simulink model "ekf_trial"  (Simulink 8.1)
settings: Solver=ode45  StartTime=0.0  StopTime=500  FixedStep=0.5  MaxStep=0.01  RelTol=1e-3
values from neighbouring files (symbols this model uses):
  A = [SUN_COPY_X,SUN_COPY_Y,SUN_COPY_Z]    [returnNormalsAndFluxes.m]
  B = [0,1,0]    [returnNormalsAndFluxes.m]
  R = [new_x;new_y;new_z]    [FINAL_PROGRAM.m]    (also in Graphical_Calculation.m; optimizedCalculation.m; optimizedCalculation_FINAL.m; returnNormalsAndFluxes.m)
undefined symbols (not defined in the file or in its folder): Ad, Bd, C, dt, L, P0_guess, Q, x0, x0_guess
settings Model: Creator=Sumeet Singh  LastModifiedBy=DJackson
settings SolverCC: ZcThreshold=1e-8  ZeroCrossControl=EnableAll  ZeroCrossAlgorithm=Adaptive
settings DataIOCC: ExternalInput=tu  LimitDataPoints=off
settings DebuggingCC: SolverPrmCheckMsg=none
settings SFSimCC: SimParseCustomCode=off

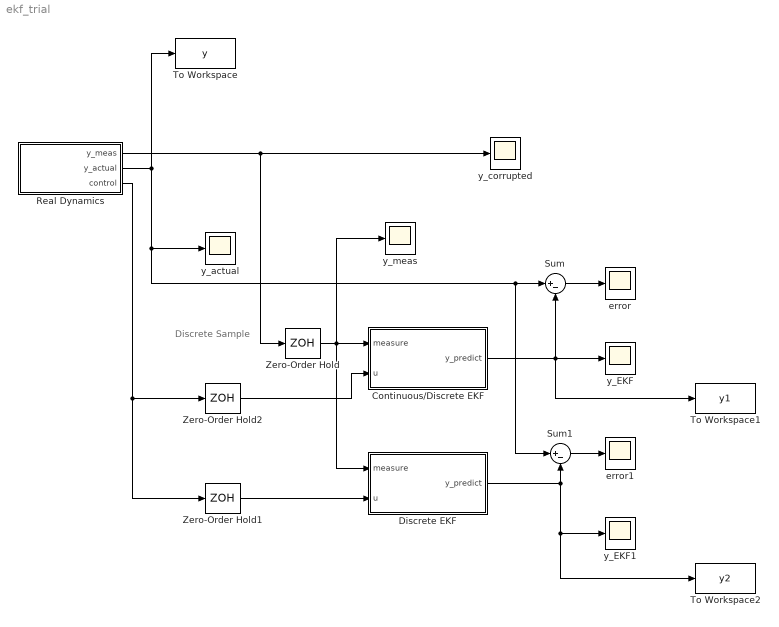
== system ekf_trial ==
  note: Discrete Sample
  Continuous/Discrete EKF : Subsystem
  Discrete EKF : Subsystem
  "Real Dynamics " : Subsystem
  Sum : Sum  Inputs=|+-
  Sum1 : Sum  Inputs=|+-
  To Workspace : ToWorkspace  VariableName=y  SampleTime=dt
  To Workspace1 : ToWorkspace  VariableName=y1  SampleTime=dt
  To Workspace2 : ToWorkspace  VariableName=y2  SampleTime=dt
  Zero-Order Hold : ZeroOrderHold  SampleTime=dt
  Zero-Order Hold1 : ZeroOrderHold  SampleTime=dt
  Zero-Order Hold2 : ZeroOrderHold  SampleTime=dt
  error : Scope
      settings: SaveName=ScopeData5
  error1 : Scope
      settings: SaveName=ScopeData6
  y_EKF : Scope
      settings: SaveName=ScopeData2
  y_EKF1 : Scope
      settings: SaveName=ScopeData8
  y_actual : Scope
  y_corrupted : Scope
  y_meas : Scope
      settings: SaveName=ScopeData4
  wires:
  Continuous/Discrete EKF/1(y_predict) -> To Workspace1/1, Sum/2, y_EKF/1
  "Real Dynamics "/3(control) -> Zero-Order Hold2/1, Zero-Order Hold1/1
  "Real Dynamics "/1(y_meas) -> y_corrupted/1, Zero-Order Hold/1
  "Real Dynamics "/2(y_actual) -> Sum1/1, Sum/1, y_actual/1, To Workspace/1
  Sum/1 -> error/1
  Zero-Order Hold1/1 -> Discrete EKF/2(u)
  Zero-Order Hold/1 -> Continuous/Discrete EKF/1(measure), y_meas/1, Discrete EKF/1(measure)
  Discrete EKF/1(y_predict) -> To Workspace2/1, y_EKF1/1, Sum1/2
  Sum1/1 -> error1/1
  Zero-Order Hold2/1 -> Continuous/Discrete EKF/2(u)

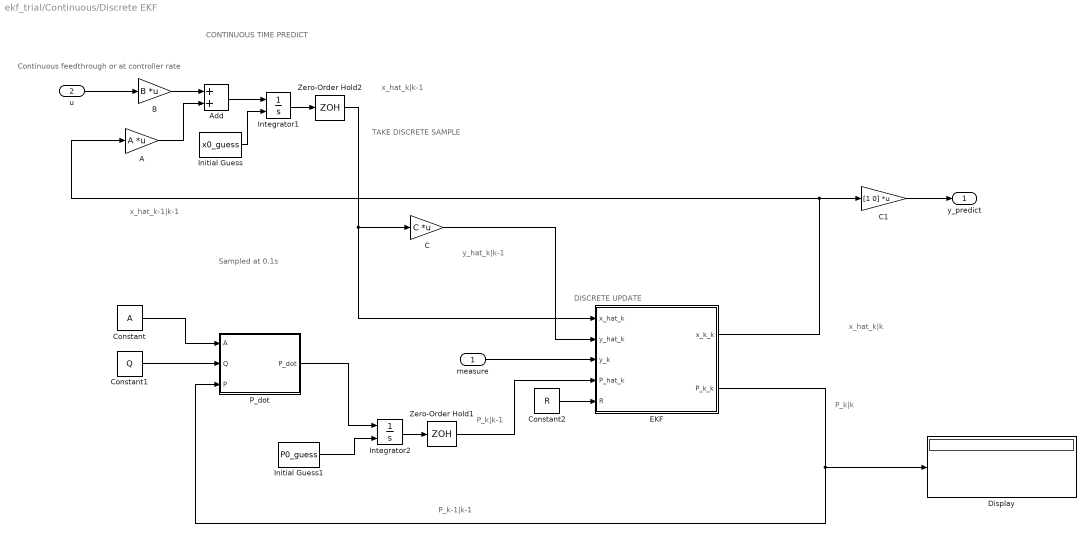
== system ekf_trial/Continuous/Discrete EKF ==
  note: TAKE DISCRETE SAMPLE
  note: x_hat_k-1|k-1
  note: x_hat_k|k-1
  note: y_hat_k|k-1
  note: DISCRETE UPDATE
  note: P_k|k-1
  note: Continuous feedthrough or at controller rate
  note: Sampled at 0.1s
  note: CONTINUOUS TIME PREDICT
  note: x_hat_k|k
  note: P_k-1|k-1
  note: P_k|k
  measure : Inport
  u : Inport  Port=2
  A : Gain  Gain=A  Multiplication=Matrix(K*u)
  Add : Sum
  B : Gain  Gain=B  Multiplication=Matrix(K*u)
  C : Gain  Gain=C  Multiplication=Matrix(K*u)
  C1 : Gain  Gain=[1 0]  Multiplication=Matrix(K*u)
  Constant : Constant  Value=A
  Constant1 : Constant  Value=Q
  Constant2 : Constant  Value=R
  Display : Display
  EKF : MATLAB Function  TreatAsAtomicUnit=on
  Initial Guess : Constant  Value=x0_guess
  Initial Guess1 : Constant  Value=P0_guess
  Integrator1 : Integrator  InitialConditionSource=external  InitialCondition=[0;20]
  Integrator2 : Integrator  InitialConditionSource=external  InitialCondition=[0;20]
  P_dot : MATLAB Function  TreatAsAtomicUnit=on
  Zero-Order Hold1 : ZeroOrderHold  SampleTime=dt
  Zero-Order Hold2 : ZeroOrderHold  SampleTime=dt
  y_predict : Outport
  wires:
  Integrator1/1 -> Zero-Order Hold2/1
  B/1 -> Add/1
  Add/1 -> Integrator1/1
  u/1 -> B/1
  C/1 -> EKF/2(y_hat_k)
  measure/1 -> EKF/3(y_k)
  Constant/1 -> P_dot/1(A)
  C1/1 -> y_predict/1
  A/1 -> Add/2
  Initial Guess/1 -> Integrator1/2
  Constant1/1 -> P_dot/2(Q)
  EKF/1(x_k_k) -> A/1, C1/1
  Constant2/1 -> EKF/5(R)
  EKF/2(P_k_k) -> P_dot/3(P), Display/1
  Zero-Order Hold1/1 -> EKF/4(P_hat_k)
  Zero-Order Hold2/1 -> EKF/1(x_hat_k), C/1
  P_dot/1(P_dot) -> Integrator2/1
  Initial Guess1/1 -> Integrator2/2
  Integrator2/1 -> Zero-Order Hold1/1

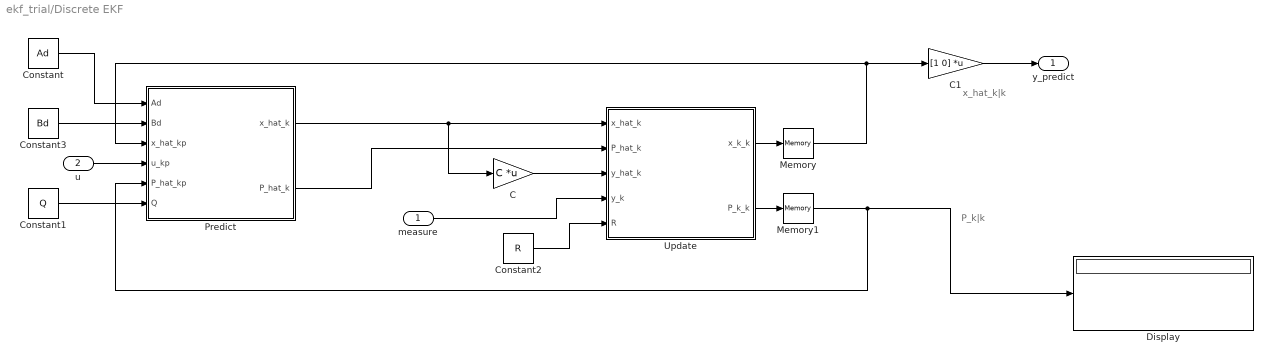
== system ekf_trial/Discrete EKF ==
  note: x_hat_k|k
  note: P_k|k
  measure : Inport
  u : Inport  Port=2
  C : Gain  Gain=C  Multiplication=Matrix(K*u)
  C1 : Gain  Gain=[1 0]  Multiplication=Matrix(K*u)
  Constant : Constant  Value=Ad
  Constant1 : Constant  Value=Q
  Constant2 : Constant  Value=R
  Constant3 : Constant  Value=Bd
  Display : Display
  Memory : Memory  X0=x0_guess  InheritSampleTime=on
  Memory1 : Memory  X0=P0_guess  InheritSampleTime=on
  Predict : MATLAB Function  TreatAsAtomicUnit=on
  Update : MATLAB Function  TreatAsAtomicUnit=on
  y_predict : Outport
  wires:
  Update/1(x_k_k) -> Memory/1
  Update/2(P_k_k) -> Memory1/1
  Constant/1 -> Predict/1(Ad)
  Constant3/1 -> Predict/2(Bd)
  u/1 -> Predict/4(u_kp)
  Constant1/1 -> Predict/6(Q)
  Predict/1(x_hat_k) -> C/1, Update/1(x_hat_k)
  C/1 -> Update/3(y_hat_k)
  Constant2/1 -> Update/5(R)
  Predict/2(P_hat_k) -> Update/2(P_hat_k)
  C1/1 -> y_predict/1
  measure/1 -> Update/4(y_k)
  Memory/1 -> C1/1, Predict/3(x_hat_kp)
  Memory1/1 -> Predict/5(P_hat_kp), Display/1

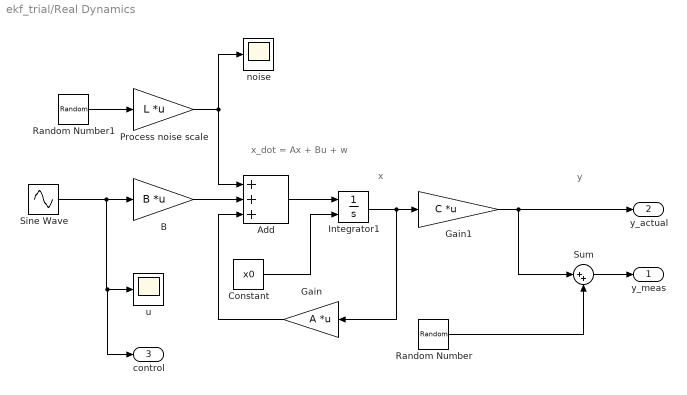
== system ekf_trial/Real Dynamics  ==
  note: y
  note: x
  note: x_dot = Ax + Bu + w
  Add : Sum  Inputs=+++
  B : Gain  Gain=B  Multiplication=Matrix(K*u)
  Constant : Constant  Value=x0
  Gain : Gain  Gain=A  Multiplication=Matrix(K*u)
  Gain1 : Gain  Gain=C  Multiplication=Matrix(K*u)
  Integrator1 : Integrator  InitialConditionSource=external
  Process noise scale : Gain  Gain=L  Multiplication=Matrix(K*u)
  Random Number : RandomNumber  Variance=R  Seed=14127  SampleTime=dt
  Random Number1 : RandomNumber  Mean=[0;0]  Seed=[6478,3164]  SampleTime=dt
  Sine Wave : Sin  Amplitude=25  Frequency=2*pi*0.5  SampleTime=0
  Sum : Sum  Inputs=|++
  noise : Scope
      settings: SaveName=ScopeData7
  u : Scope
      settings: SaveName=ScopeData3
  y_meas : Outport
  y_actual : Outport  Port=2
  control : Outport  Port=3
  wires:
  Sine Wave/1 -> control/1, u/1, B/1
  Random Number/1 -> Sum/2
  Sum/1 -> y_meas/1
  Integrator1/1 -> Gain1/1, Gain/1
  Random Number1/1 -> Process noise scale/1
  Constant/1 -> Integrator1/2
  Add/1 -> Integrator1/1
  B/1 -> Add/2
  Gain/1 -> Add/3
  Gain1/1 -> y_actual/1, Sum/1
  Process noise scale/1 -> noise/1, Add/1

== matlab function Continuous//Discrete EKF/P_dot ==
  data: A input double; Q input double; P_dot output double; P input double
function P_dot = fcn(A,Q,P)
%#coder

P_dot = A*P + P*A' + Q;

== matlab function Continuous//Discrete EKF/EKF ==
  data: x_hat_k input double; y_hat_k input double; y_k input double; x_k_k output double; P_hat_k input double; P_k_k output double; R input double
function [x_k_k, P_k_k] = fcn(x_hat_k , y_hat_k, y_k  ,P_hat_k,R)
%#coder
C = [1 0];

K = P_hat_k*C'*inv(C*P_hat_k*C' + R); %Kalman gain

x_k_k = x_hat_k + K*(y_k - y_hat_k); %Correction step for time 'k'
P_k_k = (eye(2) - K*C)*P_hat_k*(eye(2) - K*C)' + K*R*K'; % Covariance matrix update

== matlab function Discrete EKF/Update ==
  data: x_hat_k input double; P_hat_k input double; y_hat_k input double; y_k input double; x_k_k output double; P_k_k output double; R input double
function [x_k_k, P_k_k] = fcn(x_hat_k,P_hat_k,y_hat_k, y_k,R)
%#coder
C = [1 0];

K = P_hat_k*C'*inv(C*P_hat_k*C' + R); %Kalman gain

x_k_k = x_hat_k + K*(y_k - y_hat_k); %Correction step for time 'k'
% P_k_k = (eye(2) - K*C)*P_hat_k*(eye(2) - K*C)' + K*R*K'; % Covariance matrix update
P_k_k = (eye(2) - K*C)*P_hat_k;

== matlab function Discrete EKF/Predict ==
  data: x_hat_k output double; P_hat_k output double; Ad input double; Bd input double; x_hat_kp input double; u_kp input double; P_hat_kp input double; Q input double
function [x_hat_k, P_hat_k] = fcn(Ad,Bd,x_hat_kp,u_kp, P_hat_kp,Q)
%#coder

x_hat_k = Ad*x_hat_kp + Bd*u_kp;

P_hat_k = Ad*P_hat_kp*Ad' + Q;
